simulink subsystem "Localization_and_UI_Control_ThorneFleissner"  (R2020b)
settings: Solver=VariableStepAuto  StartTime=0.0  StopTime=10.0  RelTol=1e-3
settings Model: Creator=rthom  LastModifiedBy=rthom

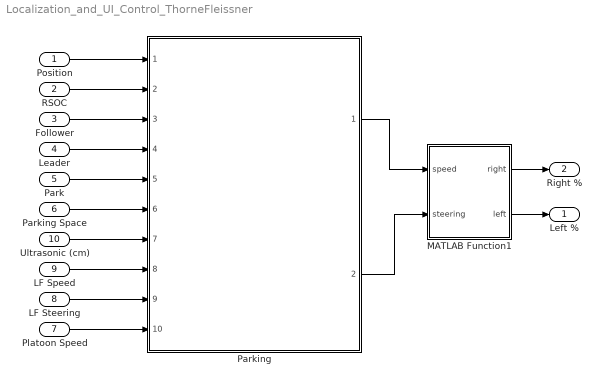
== system Localization_and_UI_Control_ThorneFleissner ==
  Position : Inport
  RSOC : Inport  Port=2
  Follower : Inport  Port=3
  Leader : Inport  Port=4
  Park : Inport  Port=5
  Parking Space : Inport  Port=6
  Platoon Speed : Inport  Port=7
  LF Steering : Inport  Port=8
  LF Speed : Inport  Port=9
  Ultrasonic (cm) : Inport  Port=10
  MATLAB Function1 : MATLAB Function  TreatAsAtomicUnit=on
  Parking : Subsystem  ReferencedSubsystem=Parking_ThorneFleissner
  Left % : Outport
  Right % : Outport  Port=2
  wires:
  LF Speed/1 -> Parking/8
  LF Steering/1 -> Parking/9
  Platoon Speed/1 -> Parking/10
  Position/1 -> Parking/1
  Ultrasonic (cm)/1 -> Parking/7
  Parking/1 -> MATLAB Function1/1(speed)
  Parking/2 -> MATLAB Function1/2(steering)
  MATLAB Function1/1(right) -> Right %/1
  MATLAB Function1/2(left) -> Left %/1
  Follower/1 -> Parking/3
  Leader/1 -> Parking/4
  Park/1 -> Parking/5
  Parking Space/1 -> Parking/6
  RSOC/1 -> Parking/2

== matlab function Localization_and_UI_Control_ThorneFleissner/MATLAB Function1 ==
  data: right output; speed input; left output; steering input
function [right, left]= toMotorSpeeds(speed, steering)

left = speed - steering;
right = speed + steering;

m = max(left,right);
if m > 100
    left = left - m + 100;
    right = right - m + 100;
end
